simulink model "aposbesh"  (R2020a)
settings: Solver=VariableStepAuto  StartTime=0.0  StopTime=100  RelTol=1e-3
settings Model: Creator=bill2  LastModifiedBy=bill2
settings DataIOCC: Refine=10

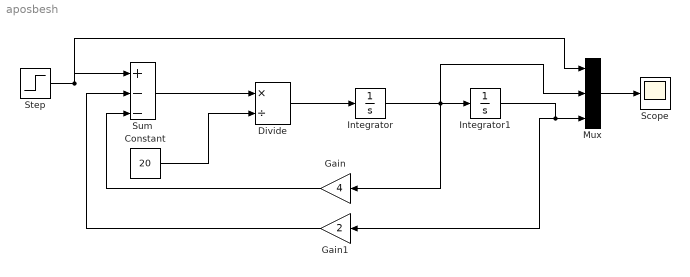
== system aposbesh ==
  Constant : Constant  Value=20
  Divide : Product  Inputs=*/
  Gain : Gain  Gain=4
  Gain1 : Gain  Gain=2
  Integrator : Integrator
  Integrator1 : Integrator  InitialCondition=4
  Mux : Mux  Inputs=3
  Scope : Scope
  Step : Step  Time=50  After=4  SampleTime=0
  Sum : Sum  Inputs=|+--
  wires:
  Step/1 -> Mux/1, Sum/1
  Sum/1 -> Divide/1
  Constant/1 -> Divide/2
  Divide/1 -> Integrator/1
  Integrator/1 -> Gain/1, Mux/2, Integrator1/1
  Integrator1/1 -> Gain1/1, Mux/3
  Gain/1 -> Sum/3
  Gain1/1 -> Sum/2
  Mux/1 -> Scope/1
